simulink model "mlf_matrix_mac"  (R2015b)
settings: Solver=ode45  StartTime=0.0  StopTime=10.0  RelTol=1e-3
libraries: dspsigattribs x4
settings Model: Creator=amatsumo  LastModifiedBy=amatsumo
settings DataIOCC: SaveFormat=Array  SignalLoggingSaveFormat=ModelDataLogs
settings OptimizationCC: BlockReduction=off  ConditionallyExecuteInputs=off  ExpressionDepthLimit=2147483647
settings DebuggingCC: UnderspecifiedInitializationDetection=Classic  MergeDetectMultiDrivingBlocksExec=none  SolverPrmCheckMsg=warning  FcnCallInpInsideContextMsg=UseLocalSettings  StateNameClashWarn=warning
settings HardwareCC: ProdBitPerPointer=32  ProdLargestAtomicFloat=None  ProdIntDivRoundTo=Undefined  ProdEndianess=Unspecified  ProdWordSize=32  ProdHWDeviceType=32-bit Generic
settings GRTTargetCC: GeneratePreprocessorConditionals=Disable all  CombineOutputUpdateFcns=off  GRTInterface=on
settings ConfigComp: CovModelRefEnable=Off  CovSFcnEnable=off

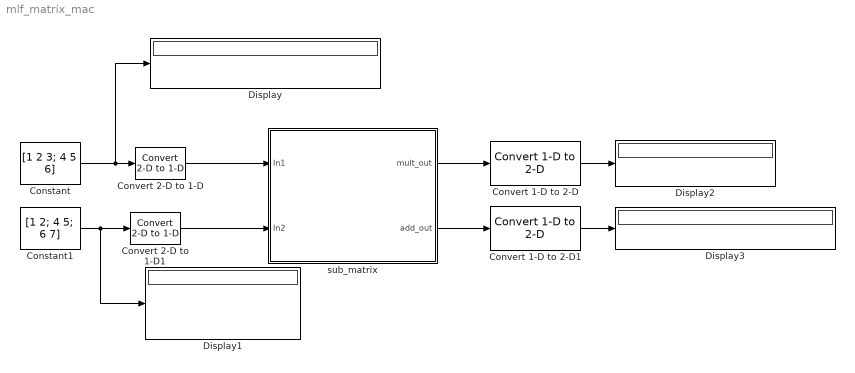
== system mlf_matrix_mac ==
  Constant : Constant  Value=[1 2 3; 4 5 6]  OutDataTypeStr=int16  SampleTime=1
  Constant1 : Constant  Value="[1 2; 4 5;  6 7]"  OutDataTypeStr=int16  SampleTime=1
  Convert 1-D to 2-D : dspsigattribs/Convert 1-D to 2-D  M=2  N=2  frameBasedOut=off
  Convert 1-D to 2-D1 : dspsigattribs/Convert 1-D to 2-D  M=2  N=3  frameBasedOut=off
  Convert 2-D to 1-D : dspsigattribs/Convert 2-D to 1-D
  Convert 2-D to 1-D1 : dspsigattribs/Convert 2-D to 1-D
  Display{,1..3} (4 alike) : Display
  sub_matrix : Subsystem
  wires:
  Constant/1 -> Convert 2-D to 1-D/1, Display/1
  Constant1/1 -> Convert 2-D to 1-D1/1, Display1/1
  Convert 2-D to 1-D/1 -> sub_matrix/1(In1)
  Convert 2-D to 1-D1/1 -> sub_matrix/2(In2)
  Convert 1-D to 2-D/1 -> Display2/1
  sub_matrix/1(mult_out) -> Convert 1-D to 2-D/1
  Convert 1-D to 2-D1/1 -> Display3/1
  sub_matrix/2(add_out) -> Convert 1-D to 2-D1/1

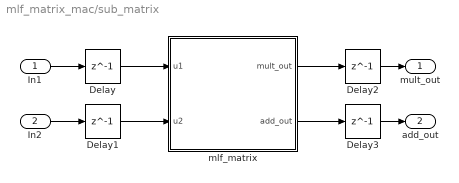
== system mlf_matrix_mac/sub_matrix ==
  In1 : Inport
  In2 : Inport  Port=2
  Delay : Delay  RequirementInfo="{}  %GIDa_6632c933_ccf5_4ee7_8d76_ef4c0c495654"  DelayLength=1
  Delay1 : Delay  RequirementInfo={} %GIDa_4709c07e_60a5_49ae_a4e8_b9deee2bd54c  DelayLength=1
  Delay2 : Delay  RequirementInfo={} %GIDa_4567d7dc_34f6_4f21_a2f7_46db77717272  DelayLength=1
  Delay3 : Delay  RequirementInfo={} %GIDa_3a899c29_6c69_4c3f_9a07_3889cee81669  DelayLength=1
  mlf_matrix : MATLAB Function  TreatAsAtomicUnit=on
  mult_out : Outport
  add_out : Outport  Port=2
  wires:
  mlf_matrix/1(mult_out) -> Delay2/1
  Delay1/1 -> mlf_matrix/2(u2)
  Delay/1 -> mlf_matrix/1(u1)
  In1/1 -> Delay/1
  In2/1 -> Delay1/1
  Delay2/1 -> mult_out/1
  Delay3/1 -> add_out/1
  mlf_matrix/2(add_out) -> Delay3/1

== matlab function mlf_matrix_mac/sub_matrix/mlf_matrix ==
  data: u1 input int16 size=6; mult_out output int16 size=4; u2 input int16 size=6; add_out output
function [mult_out,add_out] = fcn(u1, u2)
%#eml
tmp1 = reshape(u1,2,3);	% 1D=>2D
tmp2 = reshape(u2,3,2);	% 1D=>2D

tmp3 = int16(fi(tmp1,1,16,0)*fi(tmp2,1,16,0));

mult_out = tmp3(:);

tmp4 = tmp1+tmp2';

add_out = tmp4(:);
